simulink model "actual_03_discrete_estimated"  (R2024b)
settings: Solver=FixedStepDiscrete  StartTime=0.0  StopTime=10.0  FixedStep=0.1  RelTol=1e-3
settings Model: Creator=santi  LastModifiedBy=santi

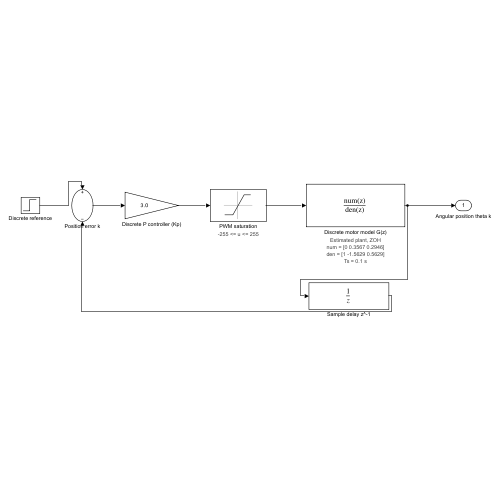
[thumbnail: Simulink's stored preview of the top-level diagram]
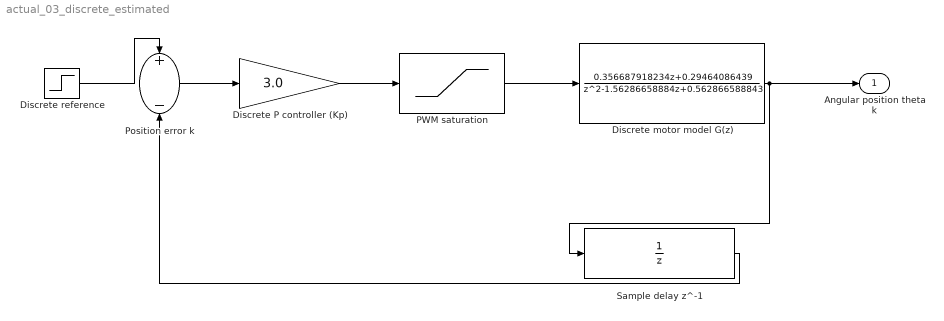
== system actual_03_discrete_estimated ==
  Discrete P controller (Kp) : Gain  Gain=3.0  SampleTime=0.1
  Discrete motor model G(z) : DiscreteTransferFcn  Numerator=[0 0.356687918234 0.29464086439]  Denominator=[1 -1.56286658884 0.562866588843]  SampleTime=0.1
      settings: AttributesFormatString=|
      | Estimated plant, ZOH
      | num = [0 0.3567 0.2946]
      | den = [1 -1.5629 0.5629]
      | Ts = 0.1 s
  Discrete reference : Step  After=45  SampleTime=0.1
  PWM saturation : Saturate  UpperLimit=255  LowerLimit=-255
      settings: AttributesFormatString=-255 <= u <= 255
  Position error k : Sum  Inputs=+-
  Sample delay z^-1 : UnitDelay  SampleTime=0.1  HasFrameUpgradeWarning=on
  Angular position theta k : Outport
  wires:
  Discrete reference/1 -> Position error k/1
  Position error k/1 -> Discrete P controller (Kp)/1
  Discrete P controller (Kp)/1 -> PWM saturation/1
  PWM saturation/1 -> Discrete motor model G(z)/1
  Discrete motor model G(z)/1 -> Angular position theta k/1, Sample delay z^-1/1
  Sample delay z^-1/1 -> Position error k/2
